simulink model "simulTP3RepRamp"  (Simulink 7.2)
settings: Solver=ode45  StartTime=0.0  StopTime=10.0  RelTol=1e-3
values from neighbouring files (symbols this model uses):
  a = -2    [SmlknValTP3Q13.m]    (also in SmlknValTP3Q14.m; SmlknValTP3Q15.m; SmlknValTP3Q16.m; simulinkValues.m)
  BE = [B E]    [SmlknValTP3Q13.m]    (also in SmlknValTP3Q14.m; SmlknValTP3Q15.m; SmlknValTP3Q16.m; simulinkValues.m)
  c = 1    [SmlknValTP3Q13.m]    (also in SmlknValTP3Q14.m; SmlknValTP3Q15.m; SmlknValTP3Q16.m; simulinkValues.m)
  d = [0 0]    [SmlknValTP3Q13.m]    (also in SmlknValTP3Q14.m; SmlknValTP3Q15.m; SmlknValTP3Q16.m; simulinkValues.m)
  Ka = acker(Aa,Ba,[-3 -3])    [SmlknValTP3Q13.m]    (also in SmlknValTP3Q14.m = acker(Aa,Ba,P); SmlknValTP3Q15.m = acker(Aa,Ba,P); SmlknValTP3Q16.m = acker(Aa,Ba,P); TP3matlabQ13.m = [k1 k2])
libraries: simulink x1
settings Model: Creator=jeremiegallee  LastModifiedBy=jeremiegallee

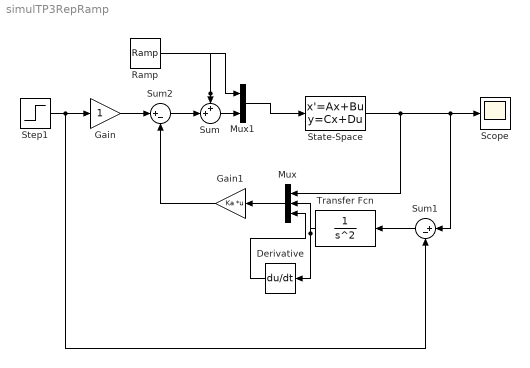
== system simulTP3RepRamp ==
  Derivative : Derivative  Orientation=left
  Gain : Gain  ParameterDataType=sfix(16)  ParameterScaling=2^0  OutDataType=sfix(16)  OutScaling=2^0
  Gain1 : Gain  Orientation=left  Gain=Ka  Multiplication=Matrix(K*u)  ParameterDataType=sfix(16)  ParameterScaling=2^0  OutDataType=sfix(16)  OutScaling=2^0
  Mux : Mux  Orientation=left  Inputs=3
  Mux1 : Mux  Inputs=2
  Ramp : simulink/Sources/Ramp  SystemSampleTime=-1  slope=1  start=0  X0=0
  Scope : Scope
  State-Space : StateSpace  A=a  B=BE  C=c  D=d
  Step1 : Step  SampleTime=0
  Sum : Sum  Inputs=++|  OutDataType=sfix(16)  OutScaling=2^0
  Sum1 : Sum  Orientation=left  Inputs=|+-  OutDataType=sfix(16)  OutScaling=2^0
  Sum2 : Sum  Inputs=|+-  OutDataType=sfix(16)  OutScaling=2^0
  Transfer Fcn : TransferFcn  Orientation=left  Denominator=[1 0 0]
  wires:
  Gain/1 -> Sum2/1
  Sum2/1 -> Sum/2
  State-Space/1 -> Mux/1, Scope/1, Sum1/1
  Mux/1 -> Gain1/1
  Gain1/1 -> Sum2/2
  Step1/1 -> Gain/1, Sum1/2
  Ramp/1 -> Mux1/1, Sum/1
  Sum/1 -> Mux1/2
  Mux1/1 -> State-Space/1
  Sum1/1 -> Transfer Fcn/1
  Transfer Fcn/1 -> Derivative/1, Mux/2
  Derivative/1 -> Mux/3
